simulink model "Non_Linear_model"  (R2025b)
settings: Solver=ode4  StartTime=0.0  StopTime=20  FixedStep=0.0005  RelTol=1e-3
InitFcn:
  | load('drone_model_parameters.mat');
values from neighbouring files (symbols this model uses):
  C1 = eye(2)    [discrete_lqr_sim.m]    (also in discrete_lqr_sim_route.m; kalman_observer.m)
  C2 = eye(4)    [discrete_lqr_sim.m]    (also in discrete_lqr_sim_route.m; kalman_observer.m)
  C3 = eye(4)    [discrete_lqr_sim.m]    (also in discrete_lqr_sim_route.m; kalman_observer.m)
  C4 = eye(2)    [discrete_lqr_sim.m]    (also in discrete_lqr_sim_route.m; kalman_observer.m)
  D1 = zeros(2, 1)    [kalman_observer.m]
  D2 = zeros(4, 1)    [kalman_observer.m]
  D3 = zeros(4, 1)    [kalman_observer.m]
  D4 = zeros(2, 1)    [kalman_observer.m]
  g = 9.81    [drone_model_parameters.mat]
  J11 = 5.8286e-05    [drone_model_parameters.mat]
  J22 = 7.1691e-05    [drone_model_parameters.mat]
  J33 = 3e-05    [drone_model_parameters.mat]
  K1 = Kd1    [discrete_lqr_sim.m]    (also in discrete_lqr_sim_route.m)
  K2 = Kd2    [discrete_lqr_sim.m]    (also in discrete_lqr_sim_route.m)
  K3 = Kd3    [discrete_lqr_sim.m]    (also in discrete_lqr_sim_route.m)
  K4 = Kd4    [discrete_lqr_sim.m]    (also in discrete_lqr_sim_route.m)
  K_T = 4.72e-08    [drone_model_parameters.mat]
  K_tau = 1.1393e-10    [drone_model_parameters.mat]
  K_u = 13840.4    [drone_model_parameters.mat]
  ki1 = 2*Kid1    [discrete_lqr_sim.m]    (also in discrete_lqr_sim_route.m)
  ki2 = 2*Kid2    [discrete_lqr_sim.m]    (also in discrete_lqr_sim_route.m)
  ki3 = Kid3    [discrete_lqr_sim.m]    (also in discrete_lqr_sim_route.m)
  ki4 = Kid4    [discrete_lqr_sim.m]    (also in discrete_lqr_sim_route.m)
  L = 0.0624    [drone_model_parameters.mat]    (also in kalman_observer.m = P * C' / R)
  m = 0.063    [drone_model_parameters.mat]
  noise_on = 1    [discrete_lqr_sim.m]    (also in discrete_lqr_sim_route.m)
  omega0 = ic(10:12)'    [discrete_lqr_sim.m]    (also in discrete_lqr_sim_route.m)
  phi_ref = 0.5    [discrete_lqr_sim.m]
  prnoise_on = 1    [discrete_lqr_sim.m]    (also in discrete_lqr_sim_route.m)
  R0_1 = R0multiplier* diag([1.8010e-3,  1.8271e-4])    [kalman_observer.m]
  R0_2 = R0multiplier* diag([4.2821e-1,  3.4817e-4,  2.2190e-3,  1.8271e-6])    [kalman_observer.m]
  R0_3 = R0multiplier* diag([7.3221e-1,  2.6060e-4,  2.2190e-3,  4.1449e-6])    [kalman_observer.m]
  r1dotguess = 0    [discrete_lqr_sim.m]    (also in discrete_lqr_sim_route.m)
  r1guess = 0    [discrete_lqr_sim.m]    (also in discrete_lqr_sim_route.m)
  r2dotguess = 0    [discrete_lqr_sim.m]    (also in discrete_lqr_sim_route.m)
  r2guess = 0    [discrete_lqr_sim.m]    (also in discrete_lqr_sim_route.m)
  r3dotguess = 0    [discrete_lqr_sim.m]    (also in discrete_lqr_sim_route.m)
  r3guess = 0    [discrete_lqr_sim.m]    (also in discrete_lqr_sim_route.m)
  r_n0 = ic(1:3)'    [discrete_lqr_sim.m]    (also in discrete_lqr_sim_route.m)
  th1dotguess = 0    [discrete_lqr_sim.m]    (also in discrete_lqr_sim_route.m)
  th1guess = 0    [discrete_lqr_sim.m]    (also in discrete_lqr_sim_route.m)
  th2dotguess = 0    [discrete_lqr_sim.m]    (also in discrete_lqr_sim_route.m)
  th2guess = 0    [discrete_lqr_sim.m]    (also in discrete_lqr_sim_route.m)
  th3dotguess = 0    [discrete_lqr_sim.m]    (also in discrete_lqr_sim_route.m)
  th3guess = 0    [discrete_lqr_sim.m]    (also in discrete_lqr_sim_route.m)
  theta0 = ic(7:9)'    [discrete_lqr_sim.m]    (also in discrete_lqr_sim_route.m)
  Ts = 0.005    [discrete_lqr_sim.m]    (also in discrete_lqr_sim_route.m)
  u_imax = 500    [drone_model_parameters.mat]
  v0 = ic(4:6)'    [discrete_lqr_sim.m]    (also in discrete_lqr_sim_route.m)
  x_ref = 1    [discrete_lqr_sim.m]
  y_ref = 2    [discrete_lqr_sim.m]
  z_ref = 4    [discrete_lqr_sim.m]
undefined symbols (not defined in the file or in its folder): Ad1, Ad2, Ad3, Ad4, Bd1, Bd2, Bd3, Bd4, DiscIntNeverNeededParam, Discrete, Kd1, Kd2, Kd3, Kd4, Kid1, Kid2, Kid3, Kid4, Time
libraries: simulink x16, ctrlSharedLib x4, matrix_library x1
settings Model: Creator=Lenovo  LastModifiedBy=joaom

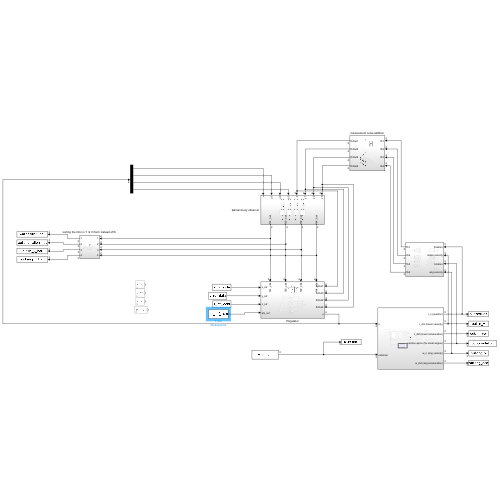
[thumbnail: Simulink's stored preview of the top-level diagram]
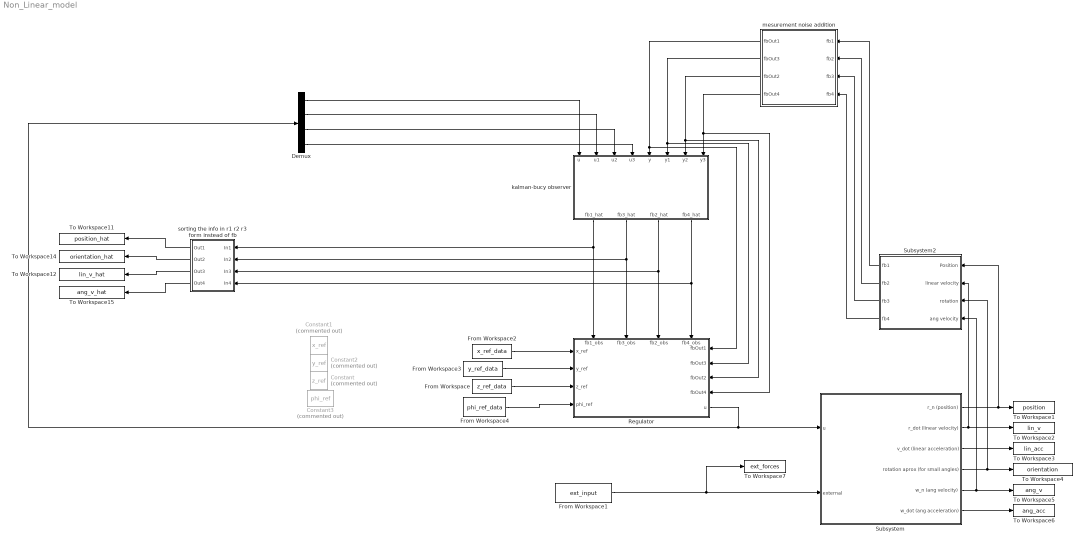
== system Non_Linear_model ==
  Constant : Constant  Commented=on  Value=z_ref
  Constant1 : Constant  Commented=on  Value=x_ref
  Constant2 : Constant  Commented=on  Value=y_ref
  Constant3 : Constant  Commented=on  Value=phi_ref
  Demux : Demux
  From Workspace : FromWorkspace  VariableName=z_ref_data  SampleTime=Ts  Interpolate=off  OutputAfterFinalValue=Holding final value
  From Workspace1 : FromWorkspace  VariableName=ext_input  SampleTime=0.01
  From Workspace2 : FromWorkspace  VariableName=x_ref_data  SampleTime=Ts  Interpolate=off  OutputAfterFinalValue=Holding final value
  From Workspace3 : FromWorkspace  VariableName=y_ref_data  SampleTime=Ts  Interpolate=off  OutputAfterFinalValue=Holding final value
  From Workspace4 : FromWorkspace  VariableName=phi_ref_data  SampleTime=Ts  Interpolate=off  OutputAfterFinalValue=Holding final value
  Regulator : Subsystem
      settings: PortSchema="{\"entries\":[{\"content\":{\"sides\":[{\"content\":{\"connectorIds\":[\"In1\",\"In2\",\"In3\",\"In4\"]},\"type\":\"ConnectorPlacement.EquallySpacedRectSide\",\"uuid\":\"b017568b-8a8c-41ec-878a-07ad52499eb1\"},{\"content\":{\"connectorIds\":[\"In9\",\"In10\",\"In11\",\"In12\",\"Out1\"],\"side\":\"RIGHT\"},\"type\":\"ConnectorPlacement.EquallySpacedRectSide\",\"uuid\":\"018e7ed3-6d8e-4146-8286-a6e4e64e27eb\"},{\"content\":{\"connectorIds\":[\"In5\",\"In6\",\"In7\",\"In8\"],\"side\":\"TOP\"},\"type\":\"ConnectorPlacement.EquallySpacedRectSide\",\"uuid\":\"74bee916-3a13-46de-9b7b-1c6e20b8f68c\"}]},\"type\":\"ConnectorPlacement.EquallySpacedConnector\",\"uuid\":\"c4290e45-5abb-401a-ab88-e47e173bbe8b\"}],\"packageUris\":[\"http://schema.mathworks.com/mf0/Connector/R2020b\"],\"version\":\"1.0\"}"
  Subsystem : Subsystem
  Subsystem2 : Subsystem
  To Workspace1 : ToWorkspace  VariableName=position  SaveFormat=Timeseries  SampleTime=-1
  To Workspace11 : ToWorkspace  VariableName=position_hat  SaveFormat=Timeseries  SampleTime=-1
  To Workspace12 : ToWorkspace  VariableName=lin_v_hat  SaveFormat=Timeseries  SampleTime=-1
  To Workspace14 : ToWorkspace  VariableName=orientation_hat  SaveFormat=Timeseries  SampleTime=-1
  To Workspace15 : ToWorkspace  VariableName=ang_v_hat  SaveFormat=Timeseries  SampleTime=-1
  To Workspace2 : ToWorkspace  VariableName=lin_v  SaveFormat=Timeseries  SampleTime=-1
  To Workspace3 : ToWorkspace  VariableName=lin_acc  SaveFormat=Timeseries  SampleTime=-1
  To Workspace4 : ToWorkspace  VariableName=orientation  SaveFormat=Timeseries  SampleTime=-1
  To Workspace5 : ToWorkspace  VariableName=ang_v  SaveFormat=Timeseries  SampleTime=-1
  To Workspace6 : ToWorkspace  VariableName=ang_acc  SaveFormat=Timeseries  SampleTime=-1
  To Workspace7 : ToWorkspace  VariableName=ext_forces  SaveFormat=Timeseries  SampleTime=-1
  kalman-bucy observer : Subsystem
  mesurement noise addition : Subsystem
  "sorting the info in r1 r2 r3 form instead of fb " : Subsystem
  wires:
  Subsystem/1(r_n (position)) -> Subsystem2/1(Position), To Workspace1/1
  From Workspace1/1 -> To Workspace7/1, Subsystem/2(external)
  Subsystem/2(r_dot (linear velocity)) -> Subsystem2/2(linear velocity), To Workspace2/1
  Subsystem/4(rotation aprox (for small angles)) -> Subsystem2/3(rotation), To Workspace4/1
  Subsystem/5(w_n (ang velocity)) -> Subsystem2/4(ang velocity), To Workspace5/1
  Subsystem/6(w_dot (ang acceleration)) -> To Workspace6/1
  Subsystem/3(v_dot (linear acceleration)) -> To Workspace3/1
  Subsystem2/1(fb1) -> mesurement noise addition/1(fb1)
  Subsystem2/4(fb4) -> mesurement noise addition/4(fb4)
  Subsystem2/2(fb2) -> mesurement noise addition/2(fb2)
  Subsystem2/3(fb3) -> mesurement noise addition/3(fb3)
  Regulator/1(u) -> Demux/1, Subsystem/1(u)
  kalman-bucy observer/2(fb3_hat) -> Regulator/6(fb3_obs), "sorting the info in r1 r2 r3 form instead of fb "/2(In2)
  kalman-bucy observer/4(fb4_hat) -> Regulator/8(fb4_obs), "sorting the info in r1 r2 r3 form instead of fb "/4(In4)
  kalman-bucy observer/1(fb1_hat) -> "sorting the info in r1 r2 r3 form instead of fb "/1(In1), Regulator/5(fb1_obs)
  kalman-bucy observer/3(fb2_hat) -> Regulator/7(fb2_obs), "sorting the info in r1 r2 r3 form instead of fb "/3(In3)
  Demux/1 -> kalman-bucy observer/1(u)
  Demux/2 -> kalman-bucy observer/2(u1)
  Demux/3 -> kalman-bucy observer/3(u2)
  Demux/4 -> kalman-bucy observer/4(u3)
  mesurement noise addition/1(fbOut1) -> Regulator/9(fbOut1), kalman-bucy observer/5(y)
  mesurement noise addition/2(fbOut3) -> kalman-bucy observer/6(y1), Regulator/10(fbOut3)
  mesurement noise addition/3(fbOut2) -> Regulator/11(fbOut2), kalman-bucy observer/7(y2)
  mesurement noise addition/4(fbOut4) -> Regulator/12(fbOut4), kalman-bucy observer/8(y3)
  "sorting the info in r1 r2 r3 form instead of fb "/1(Out1) -> To Workspace11/1
  "sorting the info in r1 r2 r3 form instead of fb "/2(Out2) -> To Workspace14/1
  "sorting the info in r1 r2 r3 form instead of fb "/3(Out3) -> To Workspace12/1
  "sorting the info in r1 r2 r3 form instead of fb "/4(Out4) -> To Workspace15/1
  From Workspace/1 -> Regulator/3(z_ref)
  From Workspace2/1 -> Regulator/1(x_ref)
  From Workspace3/1 -> Regulator/2(y_ref)
  From Workspace4/1 -> Regulator/4(phi_ref)

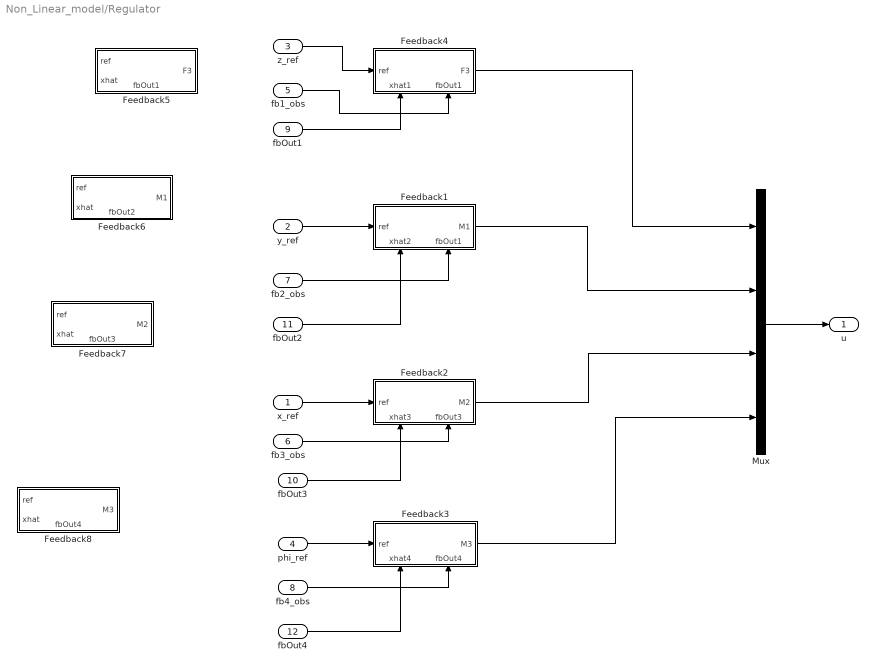
== system Non_Linear_model/Regulator ==
  x_ref : Inport
  y_ref : Inport  Port=2
  z_ref : Inport  Port=3
  phi_ref : Inport  Port=4
  fb1_obs : Inport  Port=5
  fb3_obs : Inport  Port=6
  fb2_obs : Inport  Port=7
  fb4_obs : Inport  Port=8
  fbOut1 : Inport  Port=9
  fbOut3 : Inport  Port=10
  fbOut2 : Inport  Port=11
  fbOut4 : Inport  Port=12
  Feedback1 : Subsystem
      settings: PortSchema="{\"entries\":[{\"content\":{\"sides\":[{\"content\":{\"connectorIds\":[\"In1\"]},\"type\":\"ConnectorPlacement.EquallySpacedRectSide\",\"uuid\":\"aba82e86-bea8-4dbe-bd28-9ad62cd22bb2\"},{\"content\":{\"connectorIds\":[\"Out1\"],\"side\":\"RIGHT\"},\"type\":\"ConnectorPlacement.EquallySpacedRectSide\",\"uuid\":\"b9660f25-9aef-4e33-a3fc-d60fed6e24dc\"},{\"content\":{\"side\":\"TOP\"},\"type\":\"ConnectorPlacement.EquallySpacedRectSide\",\"uuid\":\"520dc5b8-c3fb-4c94-bc3e-8116f0c42e5c\"},{\"content\":{\"connectorIds\":[\"In2\",\"In3\"],\"side\":\"BOTTOM\"},\"type\":\"ConnectorPlacement.EquallySpacedRectSide\",\"uuid\":\"509659e9-0bbe-4dc2-b074-77c88f2e837f\"}]},\"type\":\"ConnectorPlacement.EquallySpacedConnector\",\"uuid\":\"8dbbef18-a5c6-49c9-a4be-aa5f49d61e17\"}],\"packageUris\":[\"http://schema.mathworks.com/mf0/Connector/R2020b\"],\"version\":\"1.0\"}"
  Feedback2 : Subsystem
      settings: PortSchema="{\"entries\":[{\"content\":{\"sides\":[{\"content\":{\"connectorIds\":[\"In1\"]},\"type\":\"ConnectorPlacement.EquallySpacedRectSide\",\"uuid\":\"aba82e86-bea8-4dbe-bd28-9ad62cd22bb2\"},{\"content\":{\"connectorIds\":[\"Out1\"],\"side\":\"RIGHT\"},\"type\":\"ConnectorPlacement.EquallySpacedRectSide\",\"uuid\":\"b9660f25-9aef-4e33-a3fc-d60fed6e24dc\"},{\"content\":{\"side\":\"TOP\"},\"type\":\"ConnectorPlacement.EquallySpacedRectSide\",\"uuid\":\"520dc5b8-c3fb-4c94-bc3e-8116f0c42e5c\"},{\"content\":{\"connectorIds\":[\"In2\",\"In3\"],\"side\":\"BOTTOM\"},\"type\":\"ConnectorPlacement.EquallySpacedRectSide\",\"uuid\":\"509659e9-0bbe-4dc2-b074-77c88f2e837f\"}]},\"type\":\"ConnectorPlacement.EquallySpacedConnector\",\"uuid\":\"8dbbef18-a5c6-49c9-a4be-aa5f49d61e17\"}],\"packageUris\":[\"http://schema.mathworks.com/mf0/Connector/R2020b\"],\"version\":\"1.0\"}"
  Feedback3 : Subsystem
      settings: PortSchema="{\"entries\":[{\"content\":{\"sides\":[{\"content\":{\"connectorIds\":[\"In1\"]},\"type\":\"ConnectorPlacement.EquallySpacedRectSide\",\"uuid\":\"aba82e86-bea8-4dbe-bd28-9ad62cd22bb2\"},{\"content\":{\"connectorIds\":[\"Out1\"],\"side\":\"RIGHT\"},\"type\":\"ConnectorPlacement.EquallySpacedRectSide\",\"uuid\":\"b9660f25-9aef-4e33-a3fc-d60fed6e24dc\"},{\"content\":{\"side\":\"TOP\"},\"type\":\"ConnectorPlacement.EquallySpacedRectSide\",\"uuid\":\"520dc5b8-c3fb-4c94-bc3e-8116f0c42e5c\"},{\"content\":{\"connectorIds\":[\"In2\",\"In3\"],\"side\":\"BOTTOM\"},\"type\":\"ConnectorPlacement.EquallySpacedRectSide\",\"uuid\":\"509659e9-0bbe-4dc2-b074-77c88f2e837f\"}]},\"type\":\"ConnectorPlacement.EquallySpacedConnector\",\"uuid\":\"8dbbef18-a5c6-49c9-a4be-aa5f49d61e17\"}],\"packageUris\":[\"http://schema.mathworks.com/mf0/Connector/R2020b\"],\"version\":\"1.0\"}"
  Feedback4 : Subsystem
      settings: PortSchema="{\"entries\":[{\"content\":{\"sides\":[{\"content\":{\"connectorIds\":[\"In1\"]},\"type\":\"ConnectorPlacement.EquallySpacedRectSide\",\"uuid\":\"aba82e86-bea8-4dbe-bd28-9ad62cd22bb2\"},{\"content\":{\"connectorIds\":[\"Out1\"],\"side\":\"RIGHT\"},\"type\":\"ConnectorPlacement.EquallySpacedRectSide\",\"uuid\":\"b9660f25-9aef-4e33-a3fc-d60fed6e24dc\"},{\"content\":{\"side\":\"TOP\"},\"type\":\"ConnectorPlacement.EquallySpacedRectSide\",\"uuid\":\"520dc5b8-c3fb-4c94-bc3e-8116f0c42e5c\"},{\"content\":{\"connectorIds\":[\"In2\",\"In3\"],\"side\":\"BOTTOM\"},\"type\":\"ConnectorPlacement.EquallySpacedRectSide\",\"uuid\":\"509659e9-0bbe-4dc2-b074-77c88f2e837f\"}]},\"type\":\"ConnectorPlacement.EquallySpacedConnector\",\"uuid\":\"8dbbef18-a5c6-49c9-a4be-aa5f49d61e17\"}],\"packageUris\":[\"http://schema.mathworks.com/mf0/Connector/R2020b\"],\"version\":\"1.0\"}"
  Feedback5 : Subsystem
      settings: PortSchema="{\"entries\":[{\"content\":{\"sides\":[{\"content\":{\"connectorIds\":[\"In1\",\"In2\"]},\"type\":\"ConnectorPlacement.EquallySpacedRectSide\",\"uuid\":\"aba82e86-bea8-4dbe-bd28-9ad62cd22bb2\"},{\"content\":{\"connectorIds\":[\"Out1\"],\"side\":\"RIGHT\"},\"type\":\"ConnectorPlacement.EquallySpacedRectSide\",\"uuid\":\"b9660f25-9aef-4e33-a3fc-d60fed6e24dc\"},{\"content\":{\"side\":\"TOP\"},\"type\":\"ConnectorPlacement.EquallySpacedRectSide\",\"uuid\":\"520dc5b8-c3fb-4c94-bc3e-8116f0c42e5c\"},{\"content\":{\"connectorIds\":[\"In3\"],\"side\":\"BOTTOM\"},\"type\":\"ConnectorPlacement.EquallySpacedRectSide\",\"uuid\":\"509659e9-0bbe-4dc2-b074-77c88f2e837f\"}]},\"type\":\"ConnectorPlacement.EquallySpacedConnector\",\"uuid\":\"8dbbef18-a5c6-49c9-a4be-aa5f49d61e17\"}],\"packageUris\":[\"http://schema.mathworks.com/mf0/Connector/R2020b\"],\"version\":\"1.0\"}"
  Feedback6 : Subsystem
      settings: PortSchema="{\"entries\":[{\"content\":{\"sides\":[{\"content\":{\"connectorIds\":[\"In1\",\"In2\"]},\"type\":\"ConnectorPlacement.EquallySpacedRectSide\",\"uuid\":\"aba82e86-bea8-4dbe-bd28-9ad62cd22bb2\"},{\"content\":{\"connectorIds\":[\"Out1\"],\"side\":\"RIGHT\"},\"type\":\"ConnectorPlacement.EquallySpacedRectSide\",\"uuid\":\"b9660f25-9aef-4e33-a3fc-d60fed6e24dc\"},{\"content\":{\"side\":\"TOP\"},\"type\":\"ConnectorPlacement.EquallySpacedRectSide\",\"uuid\":\"520dc5b8-c3fb-4c94-bc3e-8116f0c42e5c\"},{\"content\":{\"connectorIds\":[\"In3\"],\"side\":\"BOTTOM\"},\"type\":\"ConnectorPlacement.EquallySpacedRectSide\",\"uuid\":\"a00a08e2-44b3-416a-93b7-b628ef6af78f\"}]},\"type\":\"ConnectorPlacement.EquallySpacedConnector\",\"uuid\":\"8dbbef18-a5c6-49c9-a4be-aa5f49d61e17\"}],\"packageUris\":[\"http://schema.mathworks.com/mf0/Connector/R2020b\"],\"version\":\"1.0\"}"
  Feedback7 : Subsystem
      settings: PortSchema="{\"entries\":[{\"content\":{\"sides\":[{\"content\":{\"connectorIds\":[\"In1\",\"In2\"]},\"type\":\"ConnectorPlacement.EquallySpacedRectSide\",\"uuid\":\"aba82e86-bea8-4dbe-bd28-9ad62cd22bb2\"},{\"content\":{\"connectorIds\":[\"Out1\"],\"side\":\"RIGHT\"},\"type\":\"ConnectorPlacement.EquallySpacedRectSide\",\"uuid\":\"b9660f25-9aef-4e33-a3fc-d60fed6e24dc\"},{\"content\":{\"side\":\"TOP\"},\"type\":\"ConnectorPlacement.EquallySpacedRectSide\",\"uuid\":\"520dc5b8-c3fb-4c94-bc3e-8116f0c42e5c\"},{\"content\":{\"connectorIds\":[\"In3\"],\"side\":\"BOTTOM\"},\"type\":\"ConnectorPlacement.EquallySpacedRectSide\",\"uuid\":\"6f1f9650-f53f-4fd8-a224-f107040eb56e\"}]},\"type\":\"ConnectorPlacement.EquallySpacedConnector\",\"uuid\":\"8dbbef18-a5c6-49c9-a4be-aa5f49d61e17\"}],\"packageUris\":[\"http://schema.mathworks.com/mf0/Connector/R2020b\"],\"version\":\"1.0\"}"
  Feedback8 : Subsystem
      settings: PortSchema="{\"entries\":[{\"content\":{\"sides\":[{\"content\":{\"connectorIds\":[\"In1\",\"In2\"]},\"type\":\"ConnectorPlacement.EquallySpacedRectSide\",\"uuid\":\"aba82e86-bea8-4dbe-bd28-9ad62cd22bb2\"},{\"content\":{\"connectorIds\":[\"Out1\"],\"side\":\"RIGHT\"},\"type\":\"ConnectorPlacement.EquallySpacedRectSide\",\"uuid\":\"b9660f25-9aef-4e33-a3fc-d60fed6e24dc\"},{\"content\":{\"side\":\"TOP\"},\"type\":\"ConnectorPlacement.EquallySpacedRectSide\",\"uuid\":\"520dc5b8-c3fb-4c94-bc3e-8116f0c42e5c\"},{\"content\":{\"connectorIds\":[\"In3\"],\"side\":\"BOTTOM\"},\"type\":\"ConnectorPlacement.EquallySpacedRectSide\",\"uuid\":\"cfc44da0-956d-42c7-88e2-68395bff312f\"}]},\"type\":\"ConnectorPlacement.EquallySpacedConnector\",\"uuid\":\"8dbbef18-a5c6-49c9-a4be-aa5f49d61e17\"}],\"packageUris\":[\"http://schema.mathworks.com/mf0/Connector/R2020b\"],\"version\":\"1.0\"}"
  Mux : Mux
  u : Outport
  wires:
  Feedback2/1(M2) -> Mux/3
  Feedback1/1(M1) -> Mux/2
  Feedback4/1(F3) -> Mux/1
  Feedback3/1(M3) -> Mux/4
  Mux/1 -> u/1
  x_ref/1 -> Feedback2/1(ref)
  y_ref/1 -> Feedback1/1(ref)
  z_ref/1 -> Feedback4/1(ref)
  phi_ref/1 -> Feedback3/1(ref)
  fbOut1/1 -> Feedback4/2(xhat1)
  fb1_obs/1 -> Feedback4/3(fbOut1)
  fb2_obs/1 -> Feedback1/3(fbOut1)
  fbOut2/1 -> Feedback1/2(xhat2)
  fbOut3/1 -> Feedback2/2(xhat3)
  fb3_obs/1 -> Feedback2/3(fbOut3)
  fb4_obs/1 -> Feedback3/3(fbOut4)
  fbOut4/1 -> Feedback3/2(xhat4)

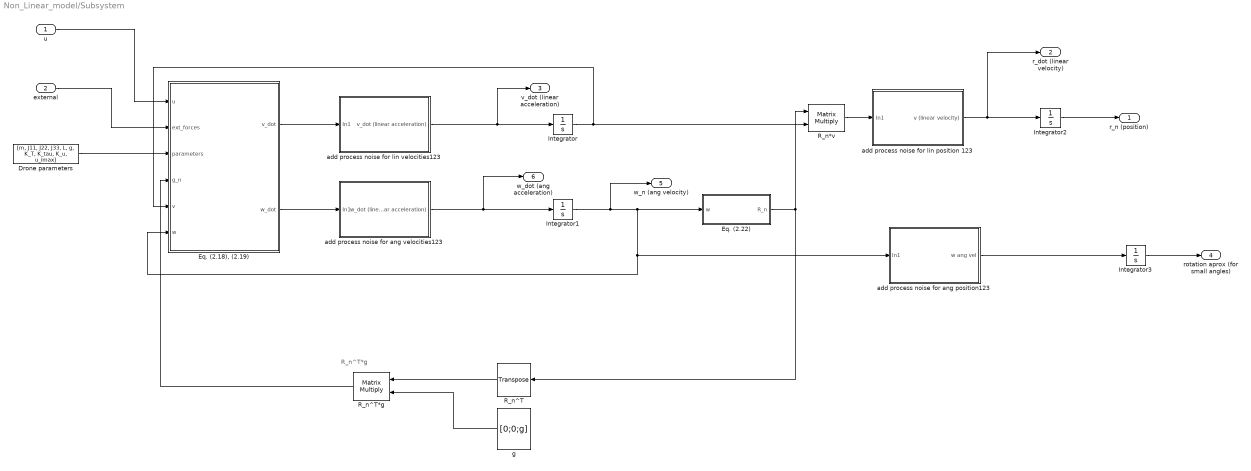
== system Non_Linear_model/Subsystem ==
  note: R_n^T*g
  u : Inport
  external : Inport  Port=2
  Drone parameters : Constant  Value=[m, J11, J22, J33, L, g, K_T, K_tau, K_u, u_imax]
  "Eq. (2.18), (2.19) " : MATLAB Function  TreatAsAtomicUnit=on
  Eq. (2.22) : Subsystem
  Integrator : Integrator  InitialCondition=v0
  Integrator1 : Integrator  InitialCondition=omega0
  Integrator2 : Integrator  InitialCondition=r_n0
  Integrator3 : Integrator  InitialCondition=theta0
  R_n*v : Product  Multiplication=Matrix(*)
  R_n^T : matrix_library/Transpose
  R_n^T*g : Product  Multiplication=Matrix(*)
  add process noise for ang position123 : Subsystem
  add process noise for ang velocities123 : Subsystem
  add process noise for lin position 123 : Subsystem
  "add process noise for lin velocities123 " : Subsystem
  g : Constant  Value=[0;0;g]  VectorParams1D=off
  r_n (position) : Outport
  r_dot (linear velocity) : Outport  Port=2
  v_dot (linear acceleration) : Outport  Port=3
  rotation aprox (for small angles) : Outport  Port=4
  w_n (ang velocity) : Outport  Port=5
  w_dot (ang acceleration) : Outport  Port=6
  wires:
  u/1 -> "Eq. (2.18), (2.19) "/1(u)
  external/1 -> "Eq. (2.18), (2.19) "/2(ext_forces)
  Drone parameters/1 -> "Eq. (2.18), (2.19) "/3(parameters)
  Eq. (2.22)/1(R_n) -> R_n*v/1, R_n^T/1
  R_n*v/1 -> add process noise for lin position 123/1(In1)
  Integrator2/1 -> r_n (position)/1
  "Eq. (2.18), (2.19) "/1(v_dot) -> "add process noise for lin velocities123 "/1(In1)
  "Eq. (2.18), (2.19) "/2(w_dot) -> add process noise for ang velocities123/1(In1)
  Integrator/1 -> "Eq. (2.18), (2.19) "/5(v), R_n*v/2
  Integrator1/1 -> w_n (ang velocity)/1, Eq. (2.22)/1(w), "Eq. (2.18), (2.19) "/6(w), add process noise for ang position123/1(In1)
  Integrator3/1 -> rotation aprox (for small angles)/1
  R_n^T/1 -> R_n^T*g/1
  g/1 -> R_n^T*g/2
  R_n^T*g/1 -> "Eq. (2.18), (2.19) "/4(g_n)
  add process noise for lin position 123/1(v (linear velocity)) -> r_dot (linear velocity)/1, Integrator2/1
  add process noise for ang position123/1(w ang vel) -> Integrator3/1
  add process noise for ang velocities123/1(w_dot (linear acceleration)) -> w_dot (ang acceleration)/1, Integrator1/1
  "add process noise for lin velocities123 "/1(v_dot (linear acceleration)) -> v_dot (linear acceleration)/1, Integrator/1

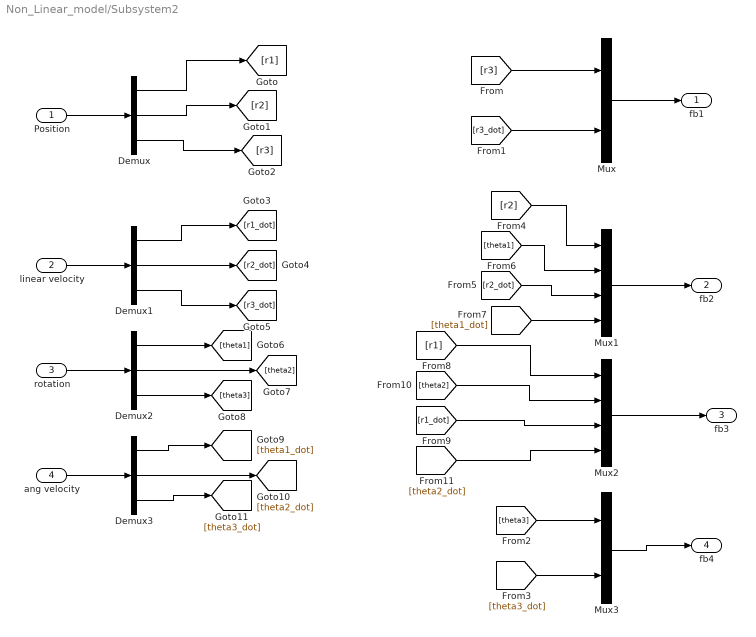
== system Non_Linear_model/Subsystem2 ==
  Position : Inport
  linear velocity : Inport  Port=2
  rotation : Inport  Port=3
  ang velocity : Inport  Port=4
  Demux{,1..3} (4 alike) : Demux  Outputs=3
  Mux : Mux  Inputs=2
  Mux1 : Mux
  Mux2 : Mux
  Mux3 : Mux  Inputs=2
  fb1 : Outport
  fb2 : Outport  Port=2
  fb3 : Outport  Port=3
  fb4 : Outport  Port=4
  wires:
  linear velocity/1 -> Demux1/1
  Position/1 -> Demux/1
  rotation/1 -> Demux2/1
  ang velocity/1 -> Demux3/1
  Demux/1 -> [r1]
  Demux/2 -> [r2]
  Demux/3 -> [r3]
  Demux1/3 -> [r3_dot]
  Demux1/1 -> [r1_dot]
  Demux1/2 -> [r2_dot]
  Demux2/3 -> [theta3]
  Demux2/2 -> [theta2]
  Demux2/1 -> [theta1]
  [r3_dot] -> Mux/2
  [r3] -> Mux/1
  Mux3/1 -> fb4/1
  Mux2/1 -> fb3/1
  Mux1/1 -> fb2/1
  Mux/1 -> fb1/1
  Demux3/3 -> [theta3_dot]
  Demux3/2 -> [theta2_dot]
  Demux3/1 -> [theta1_dot]
  [theta3_dot] -> Mux3/2
  [theta3] -> Mux3/1
  [r2] -> Mux1/1
  [r2_dot] -> Mux1/3
  [theta1] -> Mux1/2
  [theta1_dot] -> Mux1/4
  [theta2_dot] -> Mux2/4
  [r1] -> Mux2/1
  [r1_dot] -> Mux2/3
  [theta2] -> Mux2/2

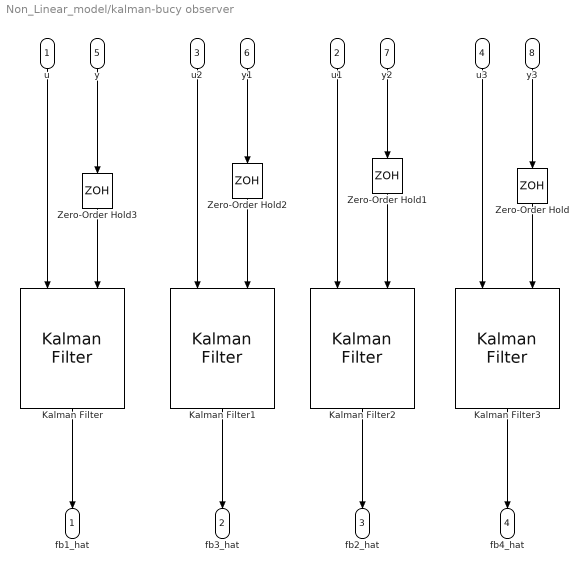
== system Non_Linear_model/kalman-bucy observer ==
  u : Inport
  u1 : Inport  Port=2
  u2 : Inport  Port=3
  u3 : Inport  Port=4
  y : Inport  Port=5
  y1 : Inport  Port=6
  y2 : Inport  Port=7
  y3 : Inport  Port=8
  Kalman Filter : ctrlSharedLib/Kalman Filter  TimeDomain=Discrete-Time  UseCurrentEstimator=on  ModelSource=Individual A, B, C, D matrices  ModelSourceVariable=ss(0.95,1,1,0,1)  A=Ad1  B=Bd1  C=C1  D=D1  NumberOfStates=1  NumberOfInputs=1  NumberOfOutputs=1  InitialEstimateSource=Dialog  X0=[r3guess; r3dotguess]  P0=10  UseK=off  UseGH=on  NumberOfProcessNoiseInputs=1  G=eye(2)  TimeInvariantG=on  H=0  TimeInvariantH=on  Q=Q0_1  TimeInvariantQ=on  R=R0_1  TimeInvariantR=on  N=0  TimeInvariantN=on  AddInputPort=on  AddEnablePort=off  OutputEstimatedY=off  OutputP=off  Ts=-1
  Kalman Filter1 : ctrlSharedLib/Kalman Filter  TimeDomain=Discrete-Time  UseCurrentEstimator=on  ModelSource=Individual A, B, C, D matrices  ModelSourceVariable=ss(0.95,1,1,0,1)  A=Ad2  B=Bd2  C=C2  D=D2  NumberOfStates=1  NumberOfInputs=1  NumberOfOutputs=1  InitialEstimateSource=Dialog  X0=[r2guess; th1guess; r2dotguess; th1dotguess]  P0=10  UseK=off  UseGH=on  NumberOfProcessNoiseInputs=1  G=eye(4)  TimeInvariantG=on  H=0  TimeInvariantH=on  Q=Q0_2  TimeInvariantQ=on  R=R0_2  TimeInvariantR=on  N=0  TimeInvariantN=on  AddInputPort=on  AddEnablePort=off  OutputEstimatedY=off  OutputP=off  Ts=-1
  Kalman Filter2 : ctrlSharedLib/Kalman Filter  TimeDomain=Discrete-Time  UseCurrentEstimator=on  ModelSource=Individual A, B, C, D matrices  ModelSourceVariable=ss(0.95,1,1,0,1)  A=Ad3  B=Bd3  C=C3  D=D3  NumberOfStates=1  NumberOfInputs=1  NumberOfOutputs=1  InitialEstimateSource=Dialog  X0=[r1guess; th2guess; r1dotguess; th2dotguess]  P0=10  UseK=off  UseGH=on  NumberOfProcessNoiseInputs=1  G=eye(4)  TimeInvariantG=on  H=0  TimeInvariantH=on  Q=Q0_3  TimeInvariantQ=on  R=R0_3  TimeInvariantR=on  N=0  TimeInvariantN=on  AddInputPort=on  AddEnablePort=off  OutputEstimatedY=off  OutputP=off  Ts=-1
  Kalman Filter3 : ctrlSharedLib/Kalman Filter  TimeDomain=Discrete-Time  UseCurrentEstimator=on  ModelSource=Individual A, B, C, D matrices  ModelSourceVariable=ss(0.95,1,1,0,1)  A=Ad4  B=Bd4  C=C4  D=D4  NumberOfStates=1  NumberOfInputs=1  NumberOfOutputs=1  InitialEstimateSource=Dialog  X0=[th3guess; th3dotguess]  P0=10  UseK=off  UseGH=on  NumberOfProcessNoiseInputs=1  G=eye(2)  TimeInvariantG=on  H=0  TimeInvariantH=on  Q=Q0_1  TimeInvariantQ=on  R=R0_1  TimeInvariantR=on  N=0  TimeInvariantN=on  AddInputPort=on  AddEnablePort=off  OutputEstimatedY=off  OutputP=off  Ts=-1
  Zero-Order Hold{,1..3} (4 alike) : ZeroOrderHold  SampleTime=Ts
  fb1_hat : Outport
  fb3_hat : Outport  Port=2
  fb2_hat : Outport  Port=3
  fb4_hat : Outport  Port=4
  wires:
  Kalman Filter/1 -> fb1_hat/1
  Kalman Filter1/1 -> fb3_hat/1
  y3/1 -> Zero-Order Hold/1
  u2/1 -> Kalman Filter1/1
  u3/1 -> Kalman Filter3/1
  Kalman Filter2/1 -> fb2_hat/1
  u1/1 -> Kalman Filter2/1
  Kalman Filter3/1 -> fb4_hat/1
  y2/1 -> Zero-Order Hold1/1
  u/1 -> Kalman Filter/1
  y1/1 -> Zero-Order Hold2/1
  y/1 -> Zero-Order Hold3/1
  Zero-Order Hold3/1 -> Kalman Filter/2
  Zero-Order Hold2/1 -> Kalman Filter1/2
  Zero-Order Hold1/1 -> Kalman Filter2/2
  Zero-Order Hold/1 -> Kalman Filter3/2

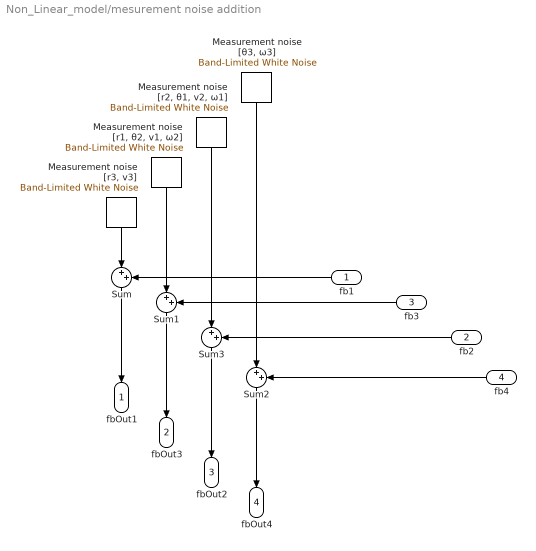
== system Non_Linear_model/mesurement noise addition ==
  fb1 : Inport
  fb2 : Inport  Port=2
  fb3 : Inport  Port=3
  fb4 : Inport  Port=4
  "Measurement noise [r1, θ2, v1, ω2] " : simulink/Sources/Band-Limited White Noise  Cov=[7.3221e-3, 2.6060e-6, 2.2190e-5, 4.1449e-8]*noise_on  Ts=0.01  seed=[23565]
  "Measurement noise [r2, θ1, v2, ω1]" : simulink/Sources/Band-Limited White Noise  Cov=[4.2821e-3, 3.4817e-6, 2.2190e-5, 1.8271e-8]*noise_on  Ts=0.01  seed=[25551]
  "Measurement noise [r3, v3]" : simulink/Sources/Band-Limited White Noise  Cov=[1.8010e-5, 1.8271e-6]*noise_on  Ts=0.01  seed=[34567]
  "Measurement noise [θ3, ω3]" : simulink/Sources/Band-Limited White Noise  Cov=[3.8313e-4, 7.0775e-8]*noise_on  Ts=0.01  seed=[44341]
  Sum{,1..3} (4 alike) : Sum  Inputs=|++
  fbOut1 : Outport
  fbOut3 : Outport  Port=2
  fbOut2 : Outport  Port=3
  fbOut4 : Outport  Port=4
  wires:
  fb4/1 -> Sum2/2
  "Measurement noise [r1, θ2, v1, ω2] "/1 -> Sum1/1
  Sum2/1 -> fbOut4/1
  fb2/1 -> Sum3/2
  Sum/1 -> fbOut1/1
  Sum1/1 -> fbOut3/1
  "Measurement noise [r2, θ1, v2, ω1]"/1 -> Sum3/1
  "Measurement noise [θ3, ω3]"/1 -> Sum2/1
  "Measurement noise [r3, v3]"/1 -> Sum/1
  Sum3/1 -> fbOut2/1
  fb1/1 -> Sum/2
  fb3/1 -> Sum1/2

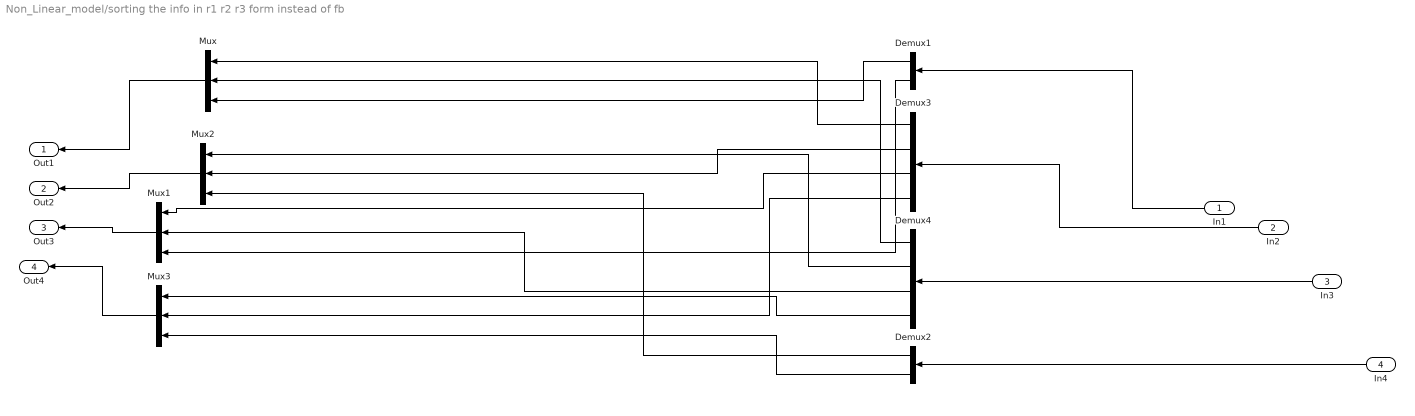
== system Non_Linear_model/sorting the info in r1 r2 r3 form instead of fb  ==
  In1 : Inport
  In2 : Inport  Port=2
  In3 : Inport  Port=3
  In4 : Inport  Port=4
  Demux1 : Demux  Outputs=2
  Demux2 : Demux  Outputs=2
  Demux3 : Demux
  Demux4 : Demux
  Mux{,1..3} (4 alike) : Mux  Inputs=3
  Out1 : Outport
  Out2 : Outport  Port=2
  Out3 : Outport  Port=3
  Out4 : Outport  Port=4
  wires:
  Demux2/2 -> Mux3/3
  Demux1/1 -> Mux/3
  Demux3/2 -> Mux2/2
  Demux4/1 -> Mux/2
  Demux2/1 -> Mux2/3
  In4/1 -> Demux2/1
  Demux4/3 -> Mux1/2
  Demux4/4 -> Mux3/1
  Demux3/1 -> Mux/1
  Demux3/4 -> Mux3/2
  Demux3/3 -> Mux1/1
  In2/1 -> Demux3/1
  Mux/1 -> Out1/1
  Demux4/2 -> Mux2/1
  Demux1/2 -> Mux1/3
  Mux3/1 -> Out4/1
  Mux2/1 -> Out2/1
  Mux1/1 -> Out3/1
  In1/1 -> Demux1/1
  In3/1 -> Demux4/1

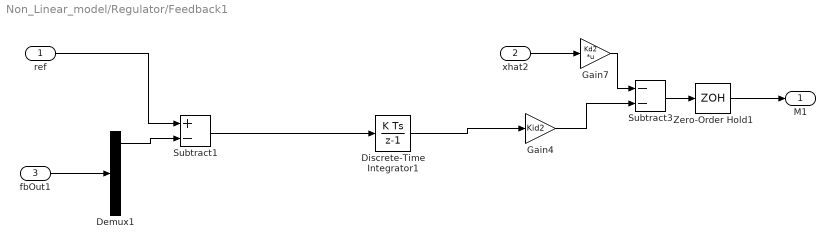
== system Non_Linear_model/Regulator/Feedback1 ==
  ref : Inport
  xhat2 : Inport  Port=2
  fbOut1 : Inport  Port=3
  Demux1 : Demux
  Discrete-Time Integrator1 : DiscreteIntegrator  SampleTime=Ts  ICPrevOutput=DiscIntNeverNeededParam  ICPrevScaledInput=DiscIntNeverNeededParam
  Gain4 : Gain  Gain=Kid2
  Gain7 : Gain  Gain=Kd2  Multiplication=Matrix(K*u)
  Subtract1 : Sum  Inputs=+-
  Subtract3 : Sum  Inputs=--
  Zero-Order Hold1 : ZeroOrderHold  SampleTime=Ts
  M1 : Outport
  wires:
  Zero-Order Hold1/1 -> M1/1
  Subtract3/1 -> Zero-Order Hold1/1
  Gain7/1 -> Subtract3/1
  Gain4/1 -> Subtract3/2
  Demux1/1 -> Subtract1/2
  fbOut1/1 -> Demux1/1
  xhat2/1 -> Gain7/1
  ref/1 -> Subtract1/1
  Subtract1/1 -> Discrete-Time Integrator1/1
  Discrete-Time Integrator1/1 -> Gain4/1

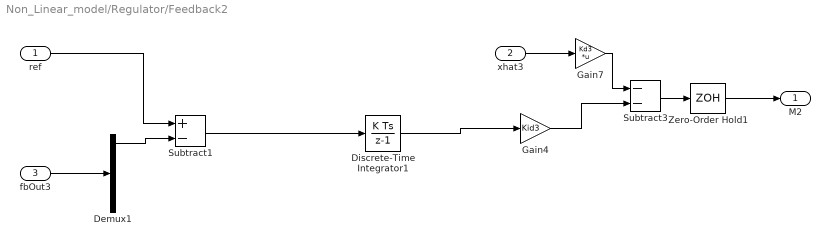
== system Non_Linear_model/Regulator/Feedback2 ==
  ref : Inport
  xhat3 : Inport  Port=2
  fbOut3 : Inport  Port=3
  Demux1 : Demux
  Discrete-Time Integrator1 : DiscreteIntegrator  SampleTime=Ts  ICPrevOutput=DiscIntNeverNeededParam  ICPrevScaledInput=DiscIntNeverNeededParam
  Gain4 : Gain  Gain=Kid3
  Gain7 : Gain  Gain=Kd3  Multiplication=Matrix(K*u)
  Subtract1 : Sum  Inputs=+-
  Subtract3 : Sum  Inputs=--
  Zero-Order Hold1 : ZeroOrderHold  SampleTime=Ts
  M2 : Outport
  wires:
  ref/1 -> Subtract1/1
  xhat3/1 -> Gain7/1
  fbOut3/1 -> Demux1/1
  Demux1/1 -> Subtract1/2
  Gain4/1 -> Subtract3/2
  Gain7/1 -> Subtract3/1
  Subtract3/1 -> Zero-Order Hold1/1
  Zero-Order Hold1/1 -> M2/1
  Subtract1/1 -> Discrete-Time Integrator1/1
  Discrete-Time Integrator1/1 -> Gain4/1

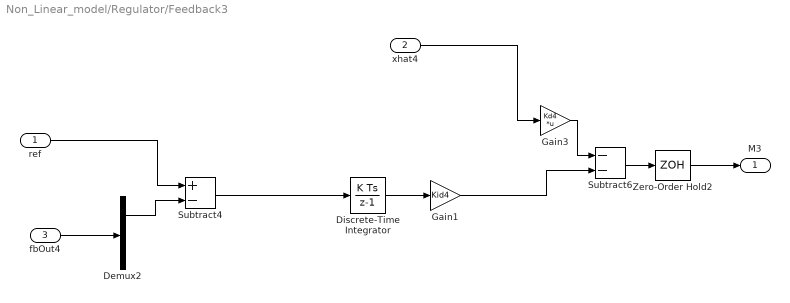
== system Non_Linear_model/Regulator/Feedback3 ==
  ref : Inport
  xhat4 : Inport  Port=2
  fbOut4 : Inport  Port=3
  Demux2 : Demux  Outputs=2
  Discrete-Time Integrator : DiscreteIntegrator  SampleTime=Ts  ICPrevOutput=DiscIntNeverNeededParam  ICPrevScaledInput=DiscIntNeverNeededParam
  Gain1 : Gain  Gain=Kid4
  Gain3 : Gain  Gain=Kd4  Multiplication=Matrix(K*u)
  Subtract4 : Sum  Inputs=+-
  Subtract6 : Sum  Inputs=--
  Zero-Order Hold2 : ZeroOrderHold  SampleTime=Ts
  M3 : Outport
  wires:
  ref/1 -> Subtract4/1
  xhat4/1 -> Gain3/1
  fbOut4/1 -> Demux2/1
  Demux2/1 -> Subtract4/2
  Gain1/1 -> Subtract6/2
  Gain3/1 -> Subtract6/1
  Subtract6/1 -> Zero-Order Hold2/1
  Zero-Order Hold2/1 -> M3/1
  Subtract4/1 -> Discrete-Time Integrator/1
  Discrete-Time Integrator/1 -> Gain1/1

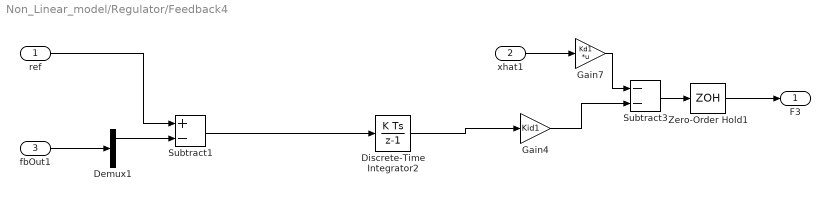
== system Non_Linear_model/Regulator/Feedback4 ==
  ref : Inport
  xhat1 : Inport  Port=2
  fbOut1 : Inport  Port=3
  Demux1 : Demux  Outputs=2
  Discrete-Time Integrator2 : DiscreteIntegrator  SampleTime=Ts  ICPrevOutput=DiscIntNeverNeededParam  ICPrevScaledInput=DiscIntNeverNeededParam
  Gain4 : Gain  Gain=Kid1
  Gain7 : Gain  Gain=Kd1  Multiplication=Matrix(K*u)
  Subtract1 : Sum  Inputs=+-
  Subtract3 : Sum  Inputs=--
  Zero-Order Hold1 : ZeroOrderHold  SampleTime=Ts
  F3 : Outport
  wires:
  ref/1 -> Subtract1/1
  xhat1/1 -> Gain7/1
  fbOut1/1 -> Demux1/1
  Demux1/1 -> Subtract1/2
  Gain4/1 -> Subtract3/2
  Gain7/1 -> Subtract3/1
  Subtract3/1 -> Zero-Order Hold1/1
  Zero-Order Hold1/1 -> F3/1
  Subtract1/1 -> Discrete-Time Integrator2/1
  Discrete-Time Integrator2/1 -> Gain4/1

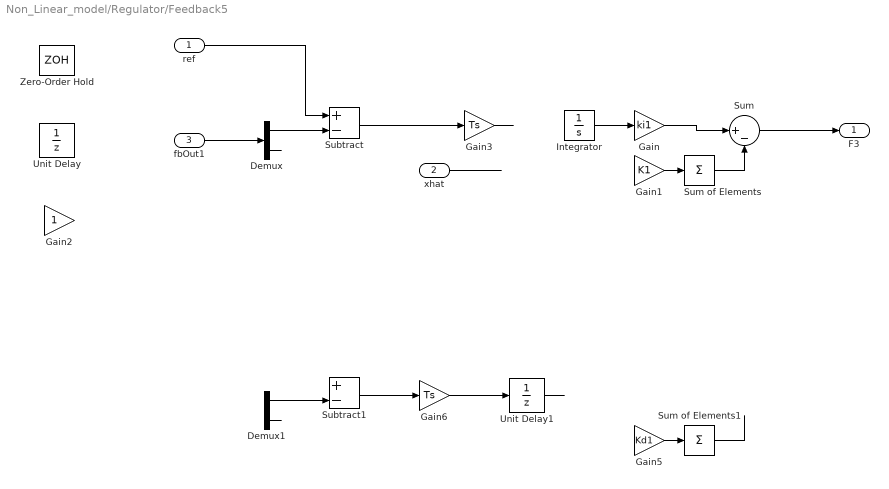
== system Non_Linear_model/Regulator/Feedback5 ==
  ref : Inport
  xhat : Inport  Port=2
  fbOut1 : Inport  Port=3
  Demux : Demux  Outputs=2
  Demux1 : Demux  Outputs=2
  Gain : Gain  Gain=ki1
  Gain1 : Gain  Gain=K1
  Gain2 : Gain
  Gain3 : Gain  Gain=Ts
  Gain5 : Gain  Gain=Kd1
  Gain6 : Gain  Gain=Ts
  Integrator : Integrator
  Subtract : Sum  Inputs=+-
  Subtract1 : Sum  Inputs=+-
  Sum : Sum  Inputs=|+-
  Sum of Elements : Sum  Inputs=+
  Sum of Elements1 : Sum  Inputs=+
  Unit Delay : UnitDelay  SampleTime=Ts  HasFrameUpgradeWarning=on
  Unit Delay1 : UnitDelay  SampleTime=Ts  HasFrameUpgradeWarning=on
  Zero-Order Hold : ZeroOrderHold  SampleTime=Ts
  F3 : Outport
  wires:
  Unit Delay1/1 -> ?
  ? -> Subtract1/1
  Gain5/1 -> Sum of Elements1/1
  ? -> ?
  ? -> ?
  Sum of Elements1/1 -> ?
  ? -> Demux1/1
  Subtract1/1 -> Gain6/1
  ? -> ?
  Demux1/2 -> ?
  Demux1/1 -> Subtract1/2
  Gain6/1 -> Unit Delay1/1
  Gain3/1 -> ?
  Demux/1 -> Subtract/2
  Demux/2 -> ?
  Integrator/1 -> Gain/1
  Subtract/1 -> Gain3/1
  fbOut1/1 -> Demux/1
  Sum of Elements/1 -> Sum/2
  Gain/1 -> Sum/1
  Sum/1 -> F3/1
  Gain1/1 -> Sum of Elements/1
  xhat/1 -> ?
  ref/1 -> Subtract/1

== system Non_Linear_model/Regulator/Feedback6 ==
  ref : Inport
  xhat : Inport  Port=2
  fbOut2 : Inport  Port=3
  Demux : Demux
  Gain : Gain  Gain=ki2
  Gain1 : Gain  Gain=K2
  Integrator : Integrator
  Subtract : Sum  Inputs=+-
  Sum : Sum  Inputs=|+-
  Sum of Elements : Sum  Inputs=+
  M1 : Outport
  wires:
  Demux/1 -> Subtract/2
  Integrator/1 -> Gain/1
  Subtract/1 -> Integrator/1
  ref/1 -> Subtract/1
  fbOut2/1 -> Demux/1
  Sum/1 -> M1/1
  Sum of Elements/1 -> Sum/2
  Gain/1 -> Sum/1
  Gain1/1 -> Sum of Elements/1
  xhat/1 -> Gain1/1

== system Non_Linear_model/Regulator/Feedback7 ==
  ref : Inport
  xhat : Inport  Port=2
  fbOut3 : Inport  Port=3
  Demux : Demux
  Gain : Gain  Gain=ki3
  Gain1 : Gain  Gain=K3
  Integrator : Integrator
  Subtract : Sum  Inputs=+-
  Sum : Sum  Inputs=|+-
  Sum of Elements : Sum  Inputs=+
  M2 : Outport
  wires:
  Integrator/1 -> Gain/1
  Demux/1 -> Subtract/2
  fbOut3/1 -> Demux/1
  ref/1 -> Subtract/1
  Subtract/1 -> Integrator/1
  Sum/1 -> M2/1
  Sum of Elements/1 -> Sum/2
  Gain/1 -> Sum/1
  Gain1/1 -> Sum of Elements/1
  xhat/1 -> Gain1/1

== system Non_Linear_model/Regulator/Feedback8 ==
  ref : Inport
  xhat : Inport  Port=2
  fbOut4 : Inport  Port=3
  Demux : Demux  Outputs=2
  Gain : Gain  Gain=ki4
  Gain1 : Gain  Gain=K4
  Integrator : Integrator
  Subtract : Sum  Inputs=+-
  Sum : Sum  Inputs=|+-
  Sum of Elements : Sum  Inputs=+
  M3 : Outport
  wires:
  Demux/1 -> Subtract/2
  Integrator/1 -> Gain/1
  Subtract/1 -> Integrator/1
  Demux/2 -> ?
  ref/1 -> Subtract/1
  fbOut4/1 -> Demux/1
  Sum/1 -> M3/1
  Sum of Elements/1 -> Sum/2
  Gain/1 -> Sum/1
  Gain1/1 -> Sum of Elements/1
  xhat/1 -> Gain1/1

== system Non_Linear_model/Subsystem/Eq. (2.22) ==
  w : Inport
  Integrator : Integrator  InitialCondition=[0;0;0]
  Matrix Multiply : Product  Multiplication=Matrix(*)
  Matrix exponential : MATLAB Function  TreatAsAtomicUnit=on
  Memory : Memory  InitialCondition=[0 0 0]
  Memory1 : Memory  InitialCondition=eye(3)
  Skew - Eq. (1.9) : MATLAB Function  TreatAsAtomicUnit=on
  Sum : Sum  Inputs=|+-
  R_n : Outport
  wires:
  w/1 -> Integrator/1
  Integrator/1 -> Memory/1, Sum/1
  Memory/1 -> Sum/2
  Sum/1 -> Skew - Eq. (1.9)/1(int_w)
  Skew - Eq. (1.9)/1(skew) -> Matrix exponential/1(skew)
  Matrix exponential/1(expM) -> Matrix Multiply/2
  Matrix Multiply/1 -> Memory1/1, R_n/1
  Memory1/1 -> Matrix Multiply/1

== system Non_Linear_model/Subsystem/add process noise for ang position123 ==
  In1 : Inport
  Demux : Demux  Outputs=3
  Mux : Mux  Inputs=3
  Sum : Sum  Inputs=|++
  Sum1 : Sum  Inputs=|++
  Sum2 : Sum  Inputs=|++
  "process noise for th1 " : simulink/Sources/Band-Limited White Noise  Cov=[0.3]*0.01*prnoise_on  Ts=0.01  seed=[84799]
  process noise for th2 : simulink/Sources/Band-Limited White Noise  Cov=[0.2]*0.01*prnoise_on  Ts=0.01  seed=[29837]
  process noise for th3 : simulink/Sources/Band-Limited White Noise  Cov=[0.1]*0.1*prnoise_on  Ts=0.01  seed=[18243]
  w ang vel : Outport
  wires:
  Mux/1 -> w ang vel/1
  In1/1 -> Demux/1
  process noise for th2/1 -> Sum1/2
  "process noise for th1 "/1 -> Sum/2
  Demux/1 -> Sum/1
  process noise for th3/1 -> Sum2/2
  Sum/1 -> Mux/1
  Sum1/1 -> Mux/2
  Sum2/1 -> Mux/3
  Demux/2 -> Sum1/1
  Demux/3 -> Sum2/1

== system Non_Linear_model/Subsystem/add process noise for ang velocities123 ==
  In1 : Inport
  Demux : Demux  Outputs=3
  Mux : Mux  Inputs=3
  Sum : Sum  Inputs=|++
  Sum1 : Sum  Inputs=|++
  Sum2 : Sum  Inputs=|++
  "process noise for w1 " : simulink/Sources/Band-Limited White Noise  Cov=[0.001]*0.01*prnoise_on  Ts=0.01  seed=[84536]
  process noise for w2 : simulink/Sources/Band-Limited White Noise  Cov=[0.001]*0.01*prnoise_on  Ts=0.01  seed=[29687]
  process noise for w3 : simulink/Sources/Band-Limited White Noise  Cov=[0.001]*0.01*prnoise_on  Ts=0.01  seed=[18383]
  w_dot (linear acceleration) : Outport
  wires:
  Mux/1 -> w_dot (linear acceleration)/1
  In1/1 -> Demux/1
  process noise for w2/1 -> Sum1/2
  "process noise for w1 "/1 -> Sum/2
  Demux/1 -> Sum/1
  process noise for w3/1 -> Sum2/2
  Sum/1 -> Mux/1
  Sum1/1 -> Mux/2
  Sum2/1 -> Mux/3
  Demux/2 -> Sum1/1
  Demux/3 -> Sum2/1

== system Non_Linear_model/Subsystem/add process noise for lin position 123 ==
  In1 : Inport
  Demux : Demux  Outputs=3
  Mux : Mux  Inputs=3
  Sum : Sum  Inputs=|++
  Sum1 : Sum  Inputs=|++
  Sum2 : Sum  Inputs=|++
  "process noise for r1 " : simulink/Sources/Band-Limited White Noise  Cov=[0.9]*0.01*prnoise_on  Ts=0.01  seed=[84766]
  process noise for r2 : simulink/Sources/Band-Limited White Noise  Cov=[0.9]*0.01*prnoise_on  Ts=0.01  seed=[29997]
  process noise for r3 : simulink/Sources/Band-Limited White Noise  Cov=[0.1]*0.01*prnoise_on  Ts=0.01  seed=[18203]
  v (linear velocity) : Outport
  wires:
  Mux/1 -> v (linear velocity)/1
  In1/1 -> Demux/1
  process noise for r2/1 -> Sum1/2
  "process noise for r1 "/1 -> Sum/2
  Demux/1 -> Sum/1
  process noise for r3/1 -> Sum2/2
  Sum/1 -> Mux/1
  Sum1/1 -> Mux/2
  Sum2/1 -> Mux/3
  Demux/2 -> Sum1/1
  Demux/3 -> Sum2/1

== system Non_Linear_model/Subsystem/add process noise for lin velocities123  ==
  In1 : Inport
  Demux : Demux  Outputs=3
  Mux : Mux  Inputs=3
  Sum : Sum  Inputs=|++
  Sum1 : Sum  Inputs=|++
  Sum2 : Sum  Inputs=|++
  process noise for 3 : simulink/Sources/Band-Limited White Noise  Cov=[0.01]*0.01*prnoise_on  Ts=0.01  seed=[18273]
  "process noise for v1 " : simulink/Sources/Band-Limited White Noise  Cov=[0.2]*0.01*prnoise_on  Ts=0.01  seed=[84736]
  process noise for v2 : simulink/Sources/Band-Limited White Noise  Cov=[0.2]*0.01*prnoise_on  Ts=0.01  seed=[29837]
  v_dot (linear acceleration) : Outport
  wires:
  Demux/3 -> Sum2/1
  Demux/2 -> Sum1/1
  Sum2/1 -> Mux/3
  Sum1/1 -> Mux/2
  Sum/1 -> Mux/1
  process noise for 3/1 -> Sum2/2
  Demux/1 -> Sum/1
  "process noise for v1 "/1 -> Sum/2
  process noise for v2/1 -> Sum1/2
  In1/1 -> Demux/1
  Mux/1 -> v_dot (linear acceleration)/1

== matlab function Non_Linear_model/Subsystem/Eq. (2.22)/Skew - Eq. (1.9) ==
  data: int_w input; skew output
function skew = fcn(int_w)

skew = [0 -int_w(3) int_w(2); int_w(3) 0 -int_w(1); -int_w(2) int_w(1) 0];

end

== matlab function Non_Linear_model/Subsystem/Eq. (2.18), (2.19)  ==
  data: u input; ext_forces input; parameters input; g_n input; v input size=3; w input size=3; v_dot output size=3; w_dot output size=3
function [v_dot, w_dot] = fcn(u, ext_forces, parameters, g_n, v, w)
% Implements Equations 2.18 and 2.19 from the quadcopter dynamics notes
%
% Inputs:
%   u           - control inputs [F3; M1; M2; M3]
%   ext_forces  - external force perturbations [F1ext; F2ext; F3ext] in body frame
%   parameters  - drone parameters [m; J11; J22; J33]
%   g_n         - gravity vector projected in body frame [g1; g2; g3]
%   v           - linear velocity in body frame [v1; v2; v3]
%   w           - angular velocity in body frame [w1; w2; w3]
%
% Outputs:
%   v_dot       - linear acceleration in body frame [v1_dot; v2_dot; v3_dot]
%   w_dot       - angular acceleration in body frame [w1_dot; w2_dot; w3_dot]

% ── Unpack parameters ─────────────────────────────────────────────────────
m   = parameters(1);
J11 = parameters(2);
J22 = parameters(3);
J33 = parameters(4);

% ── Unpack control inputs ─────────────────────────────────────────────────
F3 = u(1) - m * g_n(3);
M1 = u(2);
M2 = u(3);
M3 = u(4);

% ── Unpack external forces ────────────────────────────────────────────────
F1_ext = ext_forces(1);
F2_ext = ext_forces(2);
F3_ext = ext_forces(3);


% ── Linear acceleration - Eq. 2.18 ───────────────────────────────────────
% v_dot = Coriolis + thrust/ext forces + gravity projection
v_dot_1 = (v(2)*w(3) - v(3)*w(2)) + (F1_ext/m) + g_n(1);
v_dot_2 = (v(3)*w(1) - v(1)*w(3)) + (F2_ext/m) + g_n(2);
v_dot_3 = (v(1)*w(2) - v(2)*w(1)) + (F3/m) + (F3_ext/m) + g_n(3);

% ── Angular acceleration - Eq. 2.19 ──────────────────────────────────────
% w_dot = gyroscopic terms + applied moments
w_dot_1 = ((J22-J33)/J11) * w(2)*w(3) + M1/J11;
w_dot_2 = ((J33-J11)/J22) * w(1)*w(3) + M2/J22;
w_dot_3 = ((J11-J22)/J33) * w(1)*w(2) + M3/J33;

% ── Pack outputs ──────────────────────────────────────────────────────────
v_dot = [v_dot_1; v_dot_2; v_dot_3];
w_dot = [w_dot_1; w_dot_2; w_dot_3];

== matlab function Non_Linear_model/Subsystem/Eq. (2.22)/Matrix exponential ==
  data: skew input; expM output
function expM = fcn(skew)

expM = expm(skew);
